simulink model "AudiSim"  (R2023b)
settings: Solver=VariableStepAuto  StartTime=0.0  StopTime=7  RelTol=1e-3
values from neighbouring files (symbols this model uses):
  Crr = 65/10000    (= 0.0065)    [AudiSim_Parameters.m]
  d = 4953/10000    (= 0.4953)    [AudiSim_Parameters.m]
  g = 981/100    (= 9.81)    [AudiSim_Parameters.m]
  i = 01/10    (= 0.1)    [AudiSim_Parameters.m]
  kd = 8724/1000    (= 8.724)    [AudiSim_Parameters.m]
  m = 2145    [AudiSim_Parameters.m]
  T = 545    [AudiSim_Parameters.m]
  t_goal = 67/10    (= 6.7)    [AudiSim_Parameters.m]
  xd0 = 0    [AudiSim_Parameters.m]
  xd_goal = 277165/10000    (= 27.7165)    [AudiSim_Parameters.m]
settings Model: Creator=BeanieBabyJ  LastModifiedBy=BeanieBabyJ

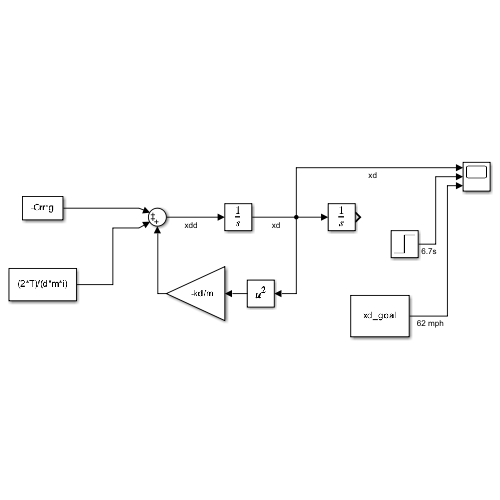
[thumbnail: Simulink's stored preview of the top-level diagram]
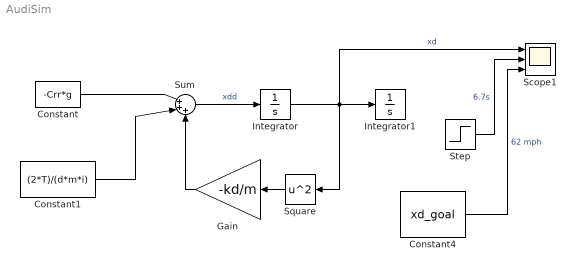
== system AudiSim ==
  Constant : Constant  Value=-Crr*g
  Constant1 : Constant  Value=(2*T)/(d*m*i)
  Constant4 : Constant  Value=xd_goal
  Gain : Gain  Gain=-kd/m
  Integrator : Integrator  InitialCondition=xd0
  Integrator1 : Integrator
  Scope1 : Scope  NumInputPorts=3
  Square : Math  Operator=square
  Step : Step  Time=t_goal  After=xd_goal  SampleTime=0
  Sum : Sum  Inputs=|+++
  wires:
  Sum/1 -> Integrator/1  "xdd"
  Square/1 -> Gain/1
  Gain/1 -> Sum/3
  Constant1/1 -> Sum/2
  Constant/1 -> Sum/1
  Step/1 -> Scope1/2  "6.7s"
  Constant4/1 -> Scope1/3  "62 mph"
  Integrator/1 -> Scope1/1, Square/1, Integrator1/1  "xd"
